simulink model "Filtro_compensa_CIC"  (R2022a)
settings: Solver=VariableStepAuto  StartTime=0.0  StopTime=sim_time  RelTol=1e-3  EnableMultiTasking=on
values from neighbouring files (symbols this model uses):
  fo = 1000    [Param_compensaCIC.m]
  fs = 50000    [Param_compensaCIC.m]
  sel_b = [0 0]    [Param_compensaCIC.m]
  Wc = 18    [Param_compensaCIC.m]
  Wc_f = 16    [Param_compensaCIC.m]
  Win = 16    [Param_compensaCIC.m]
libraries: dspsrcs4 x9
settings Model: Creator=asperez  LastModifiedBy=jose_
settings SolverCC: AlgebraicLoopSolver=TrustRegion
settings DataIOCC: ReturnWorkspaceOutputs=off
settings OptimizationCC: LifeSpan=inf
settings DebuggingCC: UnconnectedInputMsg=warning  UnconnectedOutputMsg=warning  UnconnectedLineMsg=warning  SFUnexpectedBacktrackingDiag=warning  SFNoUnconditionalDefaultTransitionDiag=warning  SFMachineParentedDataDiag=warning  ArithmeticOperatorsInVariantConditions=warning
settings SFSimCC: SimUseLocalCustomCode=off  CustomCodeUndefinedFunction=UseInterfaceOnly
settings RTWCC: RTWUseLocalCustomCode=off
settings CodeAppCC: StateflowObjectComments=on
settings GRTTargetCC: TargetLangStandard=C89/C90 (ANSI)
settings ConfigComp: CovMetricSettings=dw  CovSaveCumulativeToWorkspaceVar=on  CovSaveSingleToWorkspaceVar=on  CovExternalEMLEnable=off

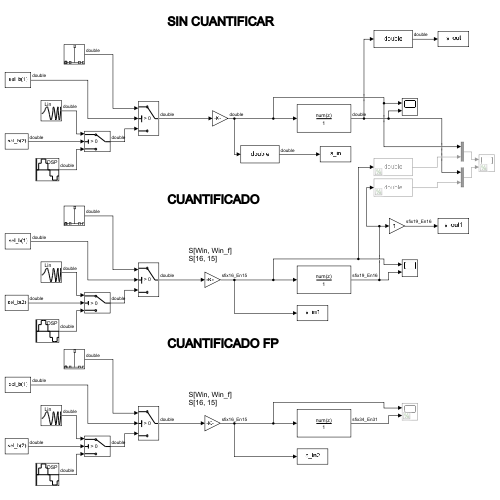
[thumbnail: Simulink's stored preview of the top-level diagram]
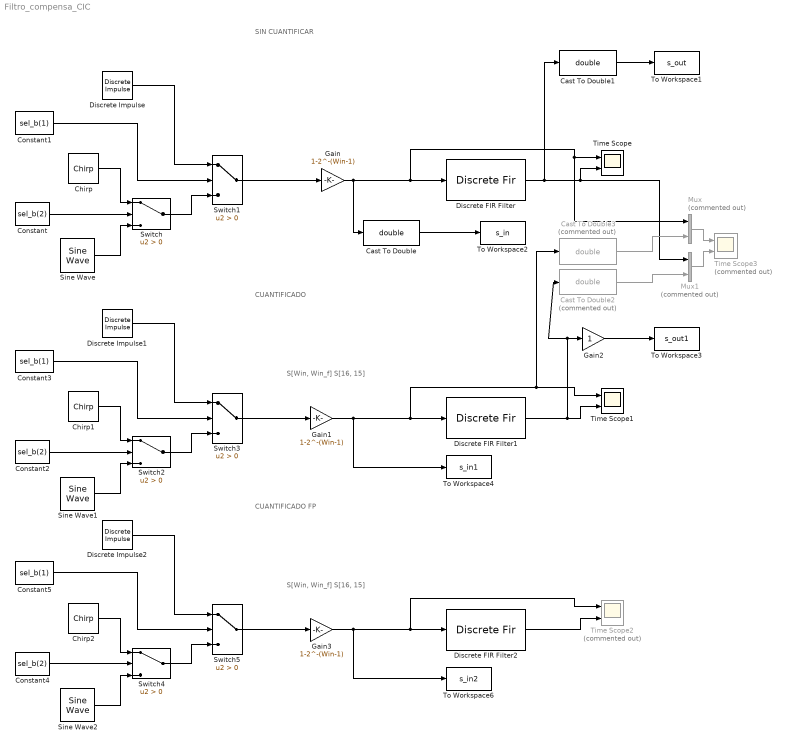
== system Filtro_compensa_CIC ==
  note: S[Win, Win_f]
      | S[16, 15]
  note: SIN CUANTIFICAR
  note: CUANTIFICADO
  note: CUANTIFICADO FP
  note: S[Win, Win_f]
      | S[16, 15]
  Cast To Double : DataTypeConversion  OutDataTypeStr=double  SaturateOnIntegerOverflow=off  RndMeth=Floor
  Cast To Double1 : DataTypeConversion  OutDataTypeStr=double  SaturateOnIntegerOverflow=off  RndMeth=Floor
  Cast To Double2 : DataTypeConversion  Commented=on  OutDataTypeStr=double  SaturateOnIntegerOverflow=off  RndMeth=Floor
  Cast To Double3 : DataTypeConversion  Commented=on  OutDataTypeStr=double  SaturateOnIntegerOverflow=off  RndMeth=Floor
  Chirp : dspsrcs4/Chirp  sweep=Linear  mode=Unidirectional  f0=1000  f1=4000  t1=1  Tsweep=1  phase=0  Ts=1/8000  spf=1  datatype=Double  OutputFrames=off
  Chirp1 : dspsrcs4/Chirp  sweep=Linear  mode=Unidirectional  f0=1000  f1=4000  t1=1  Tsweep=1  phase=0  Ts=1/8000  spf=1  datatype=Double  OutputFrames=off
  Chirp2 : dspsrcs4/Chirp  sweep=Linear  mode=Unidirectional  f0=1000  f1=4000  t1=1  Tsweep=1  phase=0  Ts=1/8000  spf=1  datatype=Double  OutputFrames=off
  Constant : Constant  Value=sel_b(2)
  Constant1 : Constant  Value=sel_b(1)
  Constant2 : Constant  Value=sel_b(2)
  Constant3 : Constant  Value=sel_b(1)
  Constant4 : Constant  Value=sel_b(2)
  Constant5 : Constant  Value=sel_b(1)
  Discrete Impulse : dspsrcs4/Discrete  Impulse  Delay=0  SampleTime=-1  FrameSample=1  OutputFrames=off  dataType=double  isSigned=on  wordLen=16  udDataType=sfix(16)  fracBitsMode=User-defined  numFracBits=15  OutDataTypeStr=double  LastOutDataTypeStr=double
  Discrete Impulse1 : dspsrcs4/Discrete  Impulse  Delay=0  SampleTime=-1  FrameSample=1  OutputFrames=off  dataType=double  isSigned=on  wordLen=16  udDataType=sfix(16)  fracBitsMode=User-defined  numFracBits=15  OutDataTypeStr=double  LastOutDataTypeStr=double
  Discrete Impulse2 : dspsrcs4/Discrete  Impulse  Delay=0  SampleTime=1/fs  FrameSample=1  OutputFrames=off  dataType=double  isSigned=on  wordLen=16  udDataType=sfix(16)  fracBitsMode=User-defined  numFracBits=15  OutDataTypeStr=double  LastOutDataTypeStr=double
  Discrete FIR Filter : DiscreteFir  Coefficients=h_q'  OutDataTypeStr=Inherit: Same as input
  Discrete FIR Filter1 : DiscreteFir  Coefficients=h_q'  CoefDataTypeStr=fixdt(1,Wc,Wc_f)  OutDataTypeStr=fixdt(1,Wout,Wout_f)
  Discrete FIR Filter2 : DiscreteFir  Coefficients=h_q'  CoefDataTypeStr=fixdt(1,Wc,Wc_f)  OutDataTypeStr=fixdt(1,34,31)
  Gain : Gain  Gain=1-2^-(Win-1)  OutDataTypeStr=double
  Gain1 : Gain  Gain=1-2^-(Win-1)  OutDataTypeStr=fixdt(1,Win,Win_f)
  Gain2 : Gain  OutDataTypeStr=fixdt(1,Wout,Wout_f)
  Gain3 : Gain  Gain=1-2^-(Win-1)  OutDataTypeStr=fixdt(1,Win,Win_f)
  Mux : Mux  Commented=on  Inputs=2
  Mux1 : Mux  Commented=on  Inputs=2
  Sine Wave : dspsrcs4/Sine Wave  Amplitude=1  Frequency=fo  Phase=0  SampleMode=Discrete  OutComplex=Real  CompMethod=Trigonometric fcn  TableSize=Speed  SampleTime=1/fs  SamplesPerFrame=1  ResetState=Restart at time zero  OutputFrames=off  dataType=double  wordLen=16  udDataType=sfix(16)  fracBitsMode=User-defined  numFracBits=14  OutDataTypeStr=double  LastOutDataTypeStr=double
  Sine Wave1 : dspsrcs4/Sine Wave  Amplitude=1  Frequency=fo  Phase=0  SampleMode=Discrete  OutComplex=Real  CompMethod=Trigonometric fcn  TableSize=Speed  SampleTime=1/fs  SamplesPerFrame=1  ResetState=Restart at time zero  OutputFrames=off  dataType=double  wordLen=16  udDataType=sfix(16)  fracBitsMode=User-defined  numFracBits=14  OutDataTypeStr=double  LastOutDataTypeStr=double
  Sine Wave2 : dspsrcs4/Sine Wave  Amplitude=1  Frequency=fo  Phase=0  SampleMode=Discrete  OutComplex=Real  CompMethod=Trigonometric fcn  TableSize=Speed  SampleTime=1/fs  SamplesPerFrame=1  ResetState=Restart at time zero  OutputFrames=off  dataType=double  wordLen=16  udDataType=sfix(16)  fracBitsMode=User-defined  numFracBits=14  OutDataTypeStr=double  LastOutDataTypeStr=double
  Switch{,1..5} (6 alike) : Switch  Criteria=u2 > Threshold  SaturateOnIntegerOverflow=off  InputSameDT=off
  Time Scope : Scope  NumInputPorts=2
  Time Scope1 : Scope  NumInputPorts=2
  Time Scope2 : Scope  Commented=on  NumInputPorts=2
  Time Scope3 : Scope  Commented=on  NumInputPorts=2
  To Workspace1 : ToWorkspace  VariableName=s_out  SampleTime=-1
  To Workspace2 : ToWorkspace  VariableName=s_in  SampleTime=-1
      settings: Save2DSignal=2-D array (concatenate along first dimension)
  To Workspace3 : ToWorkspace  VariableName=s_out1  SampleTime=-1
  To Workspace4 : ToWorkspace  VariableName=s_in1  SampleTime=-1
      settings: Save2DSignal=2-D array (concatenate along first dimension)
  To Workspace6 : ToWorkspace  VariableName=s_in2  SampleTime=-1
      settings: Save2DSignal=2-D array (concatenate along first dimension)
  wires:
  Discrete FIR Filter/1 -> Cast To Double1/1, Mux1/1, Time Scope/2
  Gain/1 -> Cast To Double/1, Mux/1, Time Scope/1, Discrete FIR Filter/1
  Cast To Double/1 -> To Workspace2/1
  Cast To Double1/1 -> To Workspace1/1
  Constant/1 -> Switch/2
  Switch/1 -> Switch1/3
  Sine Wave/1 -> Switch/3
  Constant1/1 -> Switch1/2
  Chirp/1 -> Switch/1
  Discrete Impulse/1 -> Switch1/1
  Switch1/1 -> Gain/1
  Discrete Impulse1/1 -> Switch3/1
  Chirp1/1 -> Switch2/1
  Switch3/1 -> Gain1/1
  Sine Wave1/1 -> Switch2/3
  Gain2/1 -> To Workspace3/1
  Constant2/1 -> Switch2/2
  Gain1/1 -> To Workspace4/1, Cast To Double3/1, Time Scope1/1, Discrete FIR Filter1/1
  Constant3/1 -> Switch3/2
  Switch2/1 -> Switch3/3
  Discrete FIR Filter1/1 -> Time Scope1/2, Cast To Double2/1, Gain2/1
  Constant5/1 -> Switch5/2
  Gain3/1 -> To Workspace6/1, Time Scope2/1, Discrete FIR Filter2/1
  Switch4/1 -> Switch5/3
  Switch5/1 -> Gain3/1
  Discrete FIR Filter2/1 -> Time Scope2/2
  Chirp2/1 -> Switch4/1
  Sine Wave2/1 -> Switch4/3
  Discrete Impulse2/1 -> Switch5/1
  Constant4/1 -> Switch4/2
  Mux/1 -> Time Scope3/1
  Mux1/1 -> Time Scope3/2
  Cast To Double3/1 -> Mux/2
  Cast To Double2/1 -> Mux1/2
